simulink model "mx28_identification_d"  (R2014b)
settings: Solver=FixedStepDiscrete  StartTime=0.0  StopTime=10  RelTol=1e-3
undefined symbols (not defined in the file): darwinop_communication_setup
settings Model: SimulationMode=external  Creator=florent  LastModifiedBy=florent
settings OptimizationCC: OptimizeModelRefInitCode=on  LifeSpan=1
settings HardwareCC: ProdEndianess=LittleEndian  ProdHWDeviceType=Generic->32-bit Embedded Processor
settings RTWCC: SystemTargetFile=darwinoplib.tlc  GenCodeOnly=on  TemplateMakefile=darwinoplib.tmf  Description=DarwinOP code generator  ProcessScript=darwinoplib_make_rtw_hook  TargetLang=C++
settings CodeAppCC: IgnoreCustomStorageClasses=off
settings STFCustomTargetCC: CombineOutputUpdateFcns=on  ERTCustomFileBanners=on  MatFileLogging=on  SupportContinuousTime=off  SupportNonInlinedSFcns=off  MATLABClassNameForMDSCustomization=Simulink.SoftwareTarget.ERTCustomization  GRTInterface=off  SystemTargetFile=darwinoplib.tlc
settings ERTTargetCC: ParMdlRefBuildCompliant=off  CompOptLevelCompliant=off  ConcurrentExecutionCompliant=off  ERTFirstTimeCompliant=off  MatFileLogging=on  ModelStepFunctionPrototypeControlCompliant=off  CPPClassGenCompliant=off  ExtModeStaticAlloc=on  ExtModeStaticAllocSize=100000000  ExtModeMexArgs='192.168.123.1' 1 17725  InlinedParameterPlacement=NonHierarchical  ERTCustomFileTemplate=darwinoplib_main.tlc

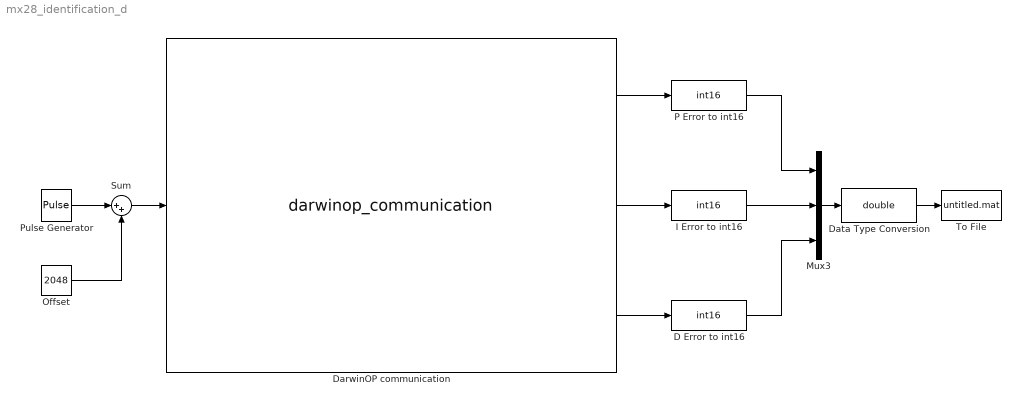
== system mx28_identification_d ==
  D Error to int16 : DataTypeConversion  OutDataTypeStr=int16  ConvertRealWorld=Stored Integer (SI)
  DarwinOP communication : M-S-Function  StartFcn=darwinop_communication_setup('StartFcn');  StopFcn=darwinop_communication_setup('StopFcn');  FunctionName=darwinop_communication  Parameters=IP,Port,Protocol,SampleTime,Frame,ReadIndex,WriteIndex  mask{IP=192.168.123.1, Port=1234, Protocol=tcp, SampleTime=0.004, Frame=[ 2 1 56 6 3 1 30 2 0 0], ReadIndex=[ 1 2;3 2;5 2], WriteIndex=[ 9 2]}
      settings: DeleteFcn=darwinop_communication_setup('DeleteFcn');  ModelCloseFcn=darwinop_communication_setup('ModelCloseFcn');  NameChangeFcn=darwinop_communication_setup('NameChangeFcn');  OpenFcn=darwinop_communication_setup('OpenFcn');
      mask TypeOptions Protocol: tcp | udp
      mask Display:
      | image('darwin-blk.jpg')
      | 
      | port_label('output',1,'Épaule droite (tangage)(1)/Erreur P')
      | port_label('output',2,'Épaule droite (tangage)(1)/Erreur I')
      | port_label('output',3,'Épaule droite (tangage)(1)/Erreur D')
      | 
      | port_label('input',1,'Épaule droite (tangage)(1)/Consigne de position')
  Data Type Conversion : DataTypeConversion  OutDataTypeStr=double
  I Error to int16 : DataTypeConversion  OutDataTypeStr=int16  ConvertRealWorld=Stored Integer (SI)
  Mux3 : Mux  Inputs=3
  Offset : Constant  Value=2048
  P Error to int16 : DataTypeConversion  OutDataTypeStr=int16  ConvertRealWorld=Stored Integer (SI)
  Pulse Generator : DiscretePulseGenerator  Amplitude=1024  Period=2000  PulseWidth=1000  PhaseDelay=250  SampleTime=0.004
  Sum : Sum  Inputs=|++
  To File : ToFile  MatrixName=Data
  wires:
  Offset/1 -> Sum/2
  Pulse Generator/1 -> Sum/1
  Mux3/1 -> Data Type Conversion/1
  Data Type Conversion/1 -> To File/1
  Sum/1 -> DarwinOP communication/1
  P Error to int16/1 -> Mux3/1
  I Error to int16/1 -> Mux3/2
  D Error to int16/1 -> Mux3/3
  DarwinOP communication/1 -> P Error to int16/1
  DarwinOP communication/2 -> I Error to int16/1
  DarwinOP communication/3 -> D Error to int16/1
